simulink model "inputOutputModel"  (R2016b)
settings: Solver=VariableStepAuto  StartTime=0.0  StopTime=10.0  RelTol=1e-3
model workspace (MAT data in the model file):
  K = 2
settings Model: Creator=Lenio  LastModifiedBy=Lenio
settings DataIOCC: ExternalInput=InSig  LoadExternalInput=on  SaveFormat=Array  SignalLogging=off  DSMLogging=off

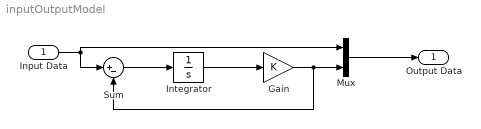
== system inputOutputModel ==
  Input Data : Inport
  Gain : Gain  Gain=K
  Integrator : Integrator
  Mux : Mux  Inputs=2
  Sum : Sum  Inputs=|+-
  Output Data : Outport
  wires:
  Input Data/1 -> Sum/1, Mux/1
  Sum/1 -> Integrator/1
  Integrator/1 -> Gain/1
  Gain/1 -> Sum/2, Mux/2
  Mux/1 -> Output Data/1
